simulink model "carsim_test2017"  (R2017b)
settings: Solver=FixedStepAuto  StartTime=0.0  StopTime=20  FixedStep=0.001  RelTol=1e-3
undefined symbols (not defined in the file or in its folder): ACC_MAP, ACC_MAP_ACCPEDL_BPY, ACC_MAP_REFSPD_BPX, BRK_MAP, BRK_MAP_BRKPEDL_BPX, ConvGear, CORNERING_STIFFNESS_APT, DIST_FR_AXLE_TO_CG_NVV, DIST_RE_AXLE_TO_CG_NVV, Fz, Fz_BPX, geartar, HYD_RATIO_APT, HYDRATIO_REFSPD_BPX, REFSPD_Q, REFSPD_R_LGT, REFSPD_R_WHL, STATIC_SPD, STATIC_TIME, VEHICLE_MASS_NVV, VEHICLE_YAW_INERTIA_NVV
libraries: simulink x22, simulink_extras x2, Solver_SF x1, SignalEditorBlockLib x1
(part 1 of 2)
settings Model: SimulationMode=accelerator  Creator=Ecoking  LastModifiedBy=Ecoking
settings DataIOCC: ReturnWorkspaceOutputs=on
settings DebuggingCC: UnconnectedInputMsg=none  UnconnectedOutputMsg=none  UnconnectedLineMsg=none
settings ModelReferenceCC: EnableRefExpFcnMdlSchedulingChecks=off
settings SFSimCC: SimUseLocalCustomCode=on
settings RTWCC: Description=Generic Real-Time Target  RTWUseLocalCustomCode=on

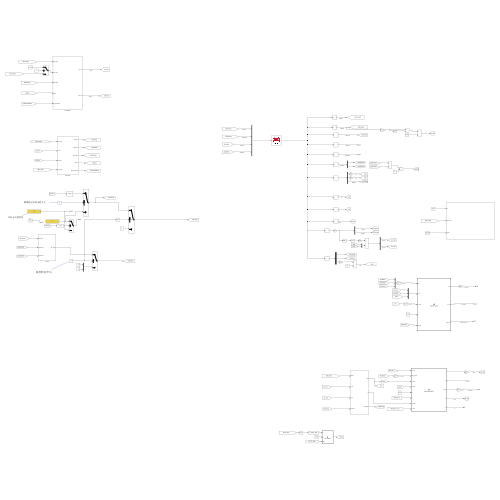
[thumbnail: Simulink's stored preview of the top-level diagram]
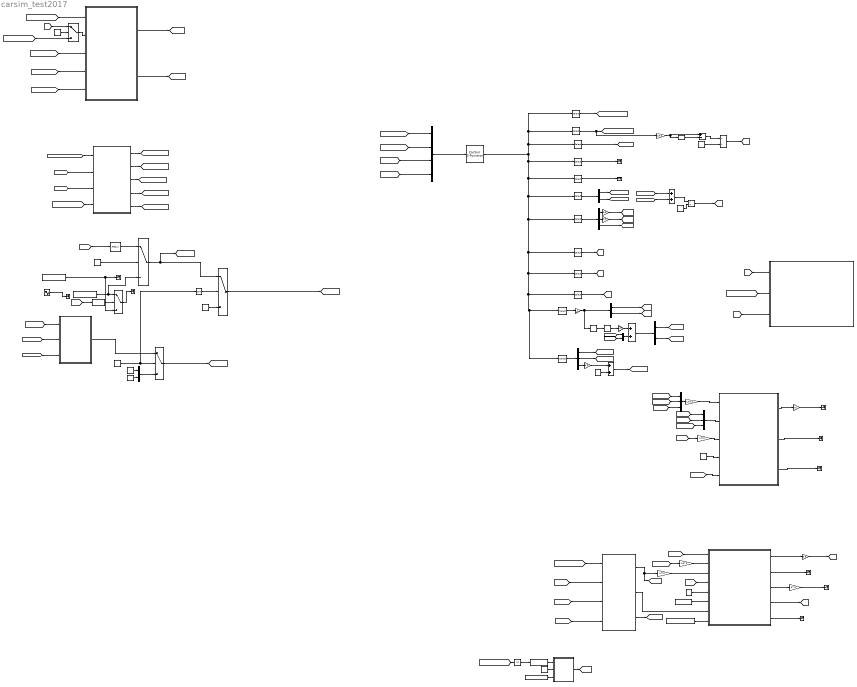
== system carsim_test2017 ==
  note: 线控转向开关
  note: 横摆稳定控制功能开关
  note: 目标方向盘转角
  Abs1 : Abs
  Add : Sum
  Add1 : Sum  Inputs=+-
  Add2 : Sum
  Add4 : Sum
  Asin : Trigonometry
  CarSim S-Function : Solver_SF/CarSim S-Function  Priority=1  SIMFILE=simfile.sim  Run_RTs=off  vs_state_ind=Run  StopMode_ind=Vehicle Model
  Compare To Constant2 : simulink/Logic and Bit Operations/Compare To Constant  relop=<=  const=STATIC_SPD  OutDataTypeStr=boolean
  Compare To Constant3 : simulink/Logic and Bit Operations/Compare To Constant  relop=<=  const=0.01  OutDataTypeStr=boolean
  Constant : Constant  Value=2
  Constant{1,11..14,25..26} (7 alike) : Constant  Value=0
  Constant{3,6..7,15} (4 alike) : Constant  Value=0.001
  Constant2 : Constant  Value=50
  Constant23 : Constant  Value=STATIC_TIME
  Constant24 : Constant  Value=REFSPD_R_LGT
  Constant4 : Constant  Value=REFSPD_Q
  Constant5 : Constant  Value=9.8
  Degrees to Radians : simulink_extras/Transformations/Degrees to Radians
  Delay : Delay  SampleTime=0.001
  Demux : Demux  Outputs=2
  Demux1 : Demux  Outputs=3
  Demux2 : Demux  Outputs=3
  Demux3 : Demux  Outputs=2
  Demux4 : Demux  Outputs=2
  Divide : Product  Inputs=*/
  Divide1 : Product  Inputs=*/
  Drv & Brk : Subsystem
  Gain{,1,6,9} (4 alike) : Gain  Gain=9.8
  Gain10 : Gain  Gain=1/3.6
  Gain11 : Gain  Gain=3.6
  Gain12 : Gain  Gain=1/57.3
  Gain2 : Gain  Gain=1/3.6
  Gain3 : Gain  Gain=3.6
  Gain4 : Gain  Gain=1/3.6
  Gain5 : Gain  Gain=-1
  Gain7 : Gain  Gain=57.3
  Gain8 : Gain  Gain=1/57.3
  Logical Operator : Logic  Operator=NOT  AllPortsSameDT=off  OutDataTypeStr=boolean
  MATLAB Function : MATLAB Function  TreatAsAtomicUnit=on
  MATLAB Function1 : MATLAB Function  TreatAsAtomicUnit=on
  MATLAB Function2 : MATLAB Function  TreatAsAtomicUnit=on
  Mux : Mux  Inputs=2
  Mux1 : Mux  Inputs=3
  Mux2 : Mux  Inputs=3
  Mux4 : Mux
  Mux9 : Mux  Inputs=2
  PID Controller1 : simulink/Continuous/PID Controller  Controller=PID  Form=Parallel  TimeDomain=Continuous-time  SampleTime=-1  IntegratorMethod=Forward Euler  ControllerParametersSource=internal  P=-10  I=-100  D=0  N=100  UseFilter=on  TunerSelectOption=Transfer Function Based (PID Tuner App)  InitialConditionSource=internal  InitialConditionForIntegrator=0  InitialConditionForFilter=0  DifferentiatorICPrevScaledInput=0  ExternalReset=none  TrackingMode=off  Kt=1  LimitOutput=off  UpperSaturationLimit=inf  LowerSaturationLimit=-inf  LinearizeAsGain=on  AntiWindupMode=none  Kb=1  POutMin=[]  POutMax=[]  IOutMin=[]  IOutMax=[]  DOutMin=[]  DOutMax=[]  NOutMin=[]  NOutMax=[]  SumOutMin=[]  SumOutMax=[]  SaturationOutMin=[]  SaturationOutMax=[]  PParamMin=[]  PParamMax=[]  IParamMin=[]  IParamMax=[]  DParamMin=[]  DParamMax=[]  NParamMin=[]  NParamMax=[]  KbParamMin=[]  KbParamMax=[]  KtParamMin=[]  KtParamMax=[]  KbOutMin=[]  KbOutMax=[]  KtOutMin=[]  KtOutMax=[]  IntegratorOutMin=[]  IntegratorOutMax=[]  FilterOutMin=[]  FilterOutMax=[]  SumI1OutMin=[]  SumI1OutMax=[]  SumI2OutMin=[]  SumI2OutMax=[]  SumI3OutMin=[]  SumI3OutMax=[]  SumDOutMin=[]  SumDOutMax=[]  DifferentiatorOutMin=[]  DifferentiatorOutMax=[]  FilterDiffOutCoefMin=[]  FilterDiffOutCoefMax=[]  ReciprocalOutMin=[]  ReciprocalOutMax=[]  SumDenOutMin=[]  SumDenOutMax=[]  SumNumOutMin=[]  SumNumOutMax=[]  DivideOutMin=[]  DivideOutMax=[]  IntegratorContinuousStateAttributes=''  IntegratorStateMustResolveToSignalObject=off  IntegratorRTWStateStorageClass=Auto  FilterContinuousStateAttributes=''  FilterStateMustResolveToSignalObject=off  FilterRTWStateStorageClass=Auto  InitialConditionSetting=State (most efficient)
  Selector : Selector  IndexOptions=Index vector (dialog)  Indices=1  OutputSizes=1
  Selector1 : Selector  IndexOptions=Index vector (dialog)  Indices=[2:5]  OutputSizes=1
  Selector12 : Selector  IndexOptions=Index vector (dialog)  Indices=[32 33]  OutputSizes=1
  Selector13 : Selector  IndexOptions=Index vector (dialog)  Indices=[34:36]  OutputSizes=1
  Selector2 : Selector  IndexOptions=Index vector (dialog)  Indices=[6:9]  OutputSizes=1
  Selector3 : Selector  IndexOptions=Index vector (dialog)  Indices=[10:13]  OutputSizes=1
  Selector4 : Selector  IndexOptions=Index vector (dialog)  Indices=[18:19]  OutputSizes=1
  Selector5 : Selector  IndexOptions=Index vector (dialog)  Indices=[20:22]  OutputSizes=1
  Selector6 : Selector  IndexOptions=Index vector (dialog)  Indices=[14:17]  OutputSizes=1
  Selector7 : Selector  IndexOptions=Index vector (dialog)  Indices=[23:26]  OutputSizes=1
  Selector8 : Selector  IndexOptions=Index vector (dialog)  Indices=[27:30]  OutputSizes=1
  Selector9 : Selector  IndexOptions=Index vector (dialog)  Indices=31  OutputSizes=1
  Sine Wave : Sin  Amplitude=50  SampleTime=0
  Subsystem : Subsystem
  Subsystem1 : Subsystem
  Switch{1..2,4..5,7} (5 alike) : Switch  Criteria=u2 > Threshold
  TCS & ABS : Subsystem
  Terminator{,1..9,11} (11 alike) : Terminator
  线控转向 : Subsystem
  wires:
  CarSim S-Function/1 -> Selector5/1, Selector8/1, Selector9/1, Selector13/1, Selector12/1, Selector7/1, Selector4/1, Selector6/1, Selector3/1, Selector2/1, Selector1/1, Selector/1
  Selector1/1 -> Gain4/1, [SPD_WHL]  "SpdWhl"
  Selector2/1 -> [MotTqAct]  "MotTqAct"
  Selector3/1 -> Terminator1/1  "HydTqAct"
  Mux4/1 -> CarSim S-Function/1
  [YawRate] -> PID Controller1/1
  PID Controller1/1 -> Switch1/1
  Constant11/1 -> Logical Operator/1, Switch4/2
  Constant12/1 -> Switch2/3
  Mux9/1 -> Switch4/3
  Switch4/1 -> [AgWhlTar]
  Constant13/1 -> Mux9/1
  Constant14/1 -> Mux9/2
  [SPD_WHL] -> TCS & ABS/1(SPD_WHL)
  [SPD_VEH] -> Switch5/3
  [MotTqDmd] -> TCS & ABS/3(MotTqDmd)
  Switch2/1 -> [SteerTar]
  Logical Operator/1 -> Switch2/2
  Switch1/1 -> [SteerDmd], Switch2/1
  Constant1/1 -> Switch1/2
  Constant2/1 -> Switch7/3, Terminator3/1
  [SteerDmd] -> 线控转向/1(SteerDmd)
  线控转向/1(pid_agwhl) -> Switch4/1
  [AgWhlActFl] -> 线控转向/2(AgWhlActFl)
  [AgWhlActFr] -> 线控转向/3(AgWhlActFr)
  Selector/1 -> [SPD_VEH]  "SpdVeh"
  Selector4/1 -> Demux/1  "AgWhlAct"
  Demux/1 -> [AgWhlActFl]
  Demux/2 -> [AgWhlActFr]
  [MotTqTar] -> Mux4/1  "MotTqTar"
  Selector6/1 -> Terminator2/1  "HydPbkAct"
  TCS & ABS/1(TcsLim) -> [TcsLim]  "TcsLim"
  [TcsLim] -> Drv & Brk/2(TcsLim)
  [SPD_VEH] -> Drv & Brk/1(SPD_VEH)
  [SPD_WHL] -> Drv & Brk/4(SPD_WHL)
  [AbsLim] -> Drv & Brk/3(MabsLim)
  Drv & Brk/1(MotTqTar) -> [MotTqTar]
  [HydPbkTar] -> Mux4/2  "HydPbkTar"
  [AgWhlTar] -> Mux4/4  "AgWhlTar"
  [SteerTar] -> Mux4/3  "SteerTar"
  Drv & Brk/2(HydPbkTar) -> [HydPbkTar]
  Drv & Brk/3(MotTqDmd) -> [MotTqDmd]
  Drv & Brk/4(Rgear) -> [Rgear]
  [Rgear] -> TCS & ABS/4(Rgear)
  Drv & Brk/5(BrkTqTotalDmd) -> [BrkTqTotalDmd]
  [BrkTqTotalDmd] -> TCS & ABS/5(BrkTqTotalDmd)
  TCS & ABS/2(AbsLim) -> [AbsLim]  "AbsLim"
  Selector5/1 -> Demux1/1
  Demux1/3 -> [YawRate]  "YawRate"
  Demux1/1 -> Gain/1
  Gain/1 -> [Lgt]  "Lgt"
  Demux1/2 -> Gain1/1
  Gain1/1 -> [Lat]  "Lat"
  Selector7/1 -> [Fz]  "Fz"
  Selector8/1 -> [Fy]  "Fy"
  Selector9/1 -> [Steer]  "Steer"
  [Fz] -> Subsystem/1(Fz)
  [SPD_VEH] -> Subsystem/2(SPD_VEH)
  [AgWhlActFl] -> Add/1
  [AgWhlActFr] -> Add/2
  Add/1 -> Divide/1
  Constant/1 -> Divide/2
  Divide/1 -> [whlag]
  [whlag] -> Subsystem/3(agwhl)
  Sine Wave/1 -> Terminator4/1
  [SPD_WHL] -> Subsystem1/1(Spdwhl)
  Subsystem1/1(Spd) -> [zv], Gain2/1  "zv"
  MATLAB Function/1(v) -> Gain3/1
  MATLAB Function/5(P) -> Terminator6/1  "P"
  MATLAB Function/3(theta) -> Gain7/1
  Gain3/1 -> [v_est]  "v_est"
  Delay/1 -> Add1/2
  Add1/1 -> Divide1/1
  Constant6/1 -> Divide1/2
  Divide1/1 -> [a_whl]
  Gain4/1 -> Delay/1, Add1/1
  Selector12/1 -> Gain5/1
  Gain5/1 -> Demux3/1, Degrees to Radians/1
  Degrees to Radians/1 -> Asin/1
  Asin/1 -> Gain6/1
  Gain6/1 -> Add4/1
  [Lgt] -> Mux/1
  Add4/1 -> Demux4/1
  Gain7/1 -> Terminator7/1  "theta_est"
  Selector13/1 -> Demux2/1
  Demux2/1 -> [PitchRate]
  Demux2/2 -> [RollRate]
  [PitchRate] -> Gain8/1
  [imu_lgt] -> MATLAB Function/1(a_meas)  "za"
  Gain8/1 -> MATLAB Function/2(omega_pitch)  "zp"
  Gain2/1 -> MATLAB Function/3(v_wheel)
  Constant3/1 -> MATLAB Function/5(dt)
  MATLAB Function/2(b) -> Terminator9/1  "b"
  Constant23/1 -> MATLAB Function1/3(delay)
  Constant15/1 -> MATLAB Function1/2(Ts)
  [SPD_VEH] -> Abs1/1
  Compare To Constant2/1 -> MATLAB Function1/1(u)
  Abs1/1 -> Compare To Constant2/1
  MATLAB Function1/1(y) -> [static]
  [static] -> MATLAB Function/4(is_static)
  Constant4/1 -> MATLAB Function/6(Q)
  Constant24/1 -> MATLAB Function/8(R_accel)
  MATLAB Function/4(a) -> [a_est]  "a_est"
  [v_est] -> Switch5/1
  Switch5/1 -> TCS & ABS/2(SPD_VEH)
  Constant25/1 -> Switch5/2
  [Agroad] -> Compare To Constant3/1
  Compare To Constant3/1 -> Switch7/2
  Constant26/1 -> Switch1/3, Switch7/1
  Switch7/1 -> Terminator11/1
  Subsystem1/2(R) -> MATLAB Function/7(R_wheel)
  [a_est] -> Subsystem1/3(a_est)
  [a_whl] -> Subsystem1/2(a_whl)
  [MotTqAct] -> Subsystem1/4(MotTqAct)
  Subsystem1/3(allSlipFlag) -> [allSlipFlag]
  Demux3/1 -> [Agroad]  "Agroad"
  Demux3/2 -> [RollSlop]  "RollSlop"
  [Lat] -> Mux/2
  Mux/1 -> Add4/2
  Demux4/1 -> [imu_lgt]  "imu_lgt"
  Demux4/2 -> [imu_lat]  "imu_lat"
  Demux2/3 -> Gain9/1
  Gain9/1 -> Add2/1
  Add2/1 -> [Vert]  "Vert"
  Constant5/1 -> Add2/2
  [RollRate] -> Mux1/1
  [YawRate] -> Mux1/3
  [PitchRate] -> Mux1/2
  Mux1/1 -> Gain12/1
  Mux2/1 -> MATLAB Function2/2(accel)
  [imu_lgt] -> Mux2/1
  [imu_lat] -> Mux2/2
  [Vert] -> Mux2/3
  [zv] -> Gain10/1
  Constant7/1 -> MATLAB Function2/4(dt)
  MATLAB Function2/1(v_car) -> Gain11/1
  [allSlipFlag] -> MATLAB Function2/5(slip_flag)
  Gain10/1 -> MATLAB Function2/3(v_wheel)
  Gain11/1 -> Terminator/1  "v_est_plus"
  Gain12/1 -> MATLAB Function2/1(gyro)
  MATLAB Function2/2(a_long) -> Terminator5/1  "a_est_plus"
  MATLAB Function2/3(pitch_deg) -> Terminator8/1  "theta_est_plus"

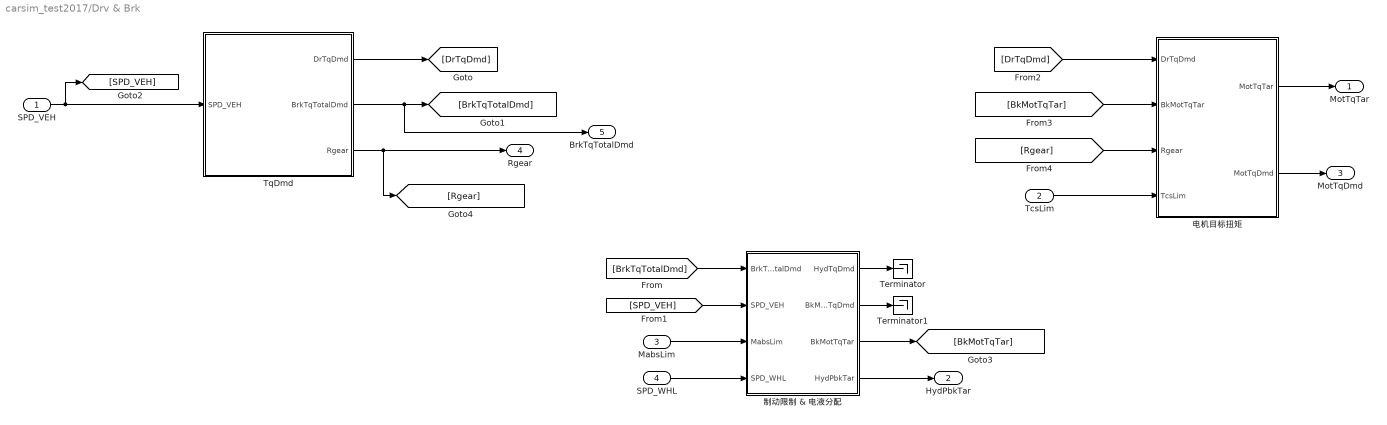
== system carsim_test2017/Drv & Brk ==
  SPD_VEH : Inport
  TcsLim : Inport  Port=2
  MabsLim : Inport  Port=3
  SPD_WHL : Inport  Port=4
  Terminator : Terminator
  Terminator1 : Terminator
  TqDmd : Subsystem
  制动限制 & 电液分配 : Subsystem
  电机目标扭矩 : Subsystem
  MotTqTar : Outport
  HydPbkTar : Outport  Port=2
  MotTqDmd : Outport  Port=3
  Rgear : Outport  Port=4
  BrkTqTotalDmd : Outport  Port=5
  wires:
  SPD_VEH/1 -> [SPD_VEH], TqDmd/1(SPD_VEH)
  TqDmd/3(Rgear) -> [Rgear], Rgear/1
  TqDmd/2(BrkTqTotalDmd) -> BrkTqTotalDmd/1, [BrkTqTotalDmd]
  TqDmd/1(DrTqDmd) -> [DrTqDmd]
  [BrkTqTotalDmd] -> 制动限制 & 电液分配/1(BrkTqTotalDmd)
  [SPD_VEH] -> 制动限制 & 电液分配/2(SPD_VEH)
  [DrTqDmd] -> 电机目标扭矩/1(DrTqDmd)
  [BkMotTqTar] -> 电机目标扭矩/2(BkMotTqTar)
  [Rgear] -> 电机目标扭矩/3(Rgear)
  TcsLim/1 -> 电机目标扭矩/4(TcsLim)
  MabsLim/1 -> 制动限制 & 电液分配/3(MabsLim)
  制动限制 & 电液分配/3(BkMotTqTar) -> [BkMotTqTar]
  SPD_WHL/1 -> 制动限制 & 电液分配/4(SPD_WHL)
  制动限制 & 电液分配/1(HydTqDmd) -> Terminator/1
  制动限制 & 电液分配/2(BkMotTqDmd) -> Terminator1/1
  制动限制 & 电液分配/4(HydPbkTar) -> HydPbkTar/1
  电机目标扭矩/1(MotTqTar) -> MotTqTar/1
  电机目标扭矩/2(MotTqDmd) -> MotTqDmd/1

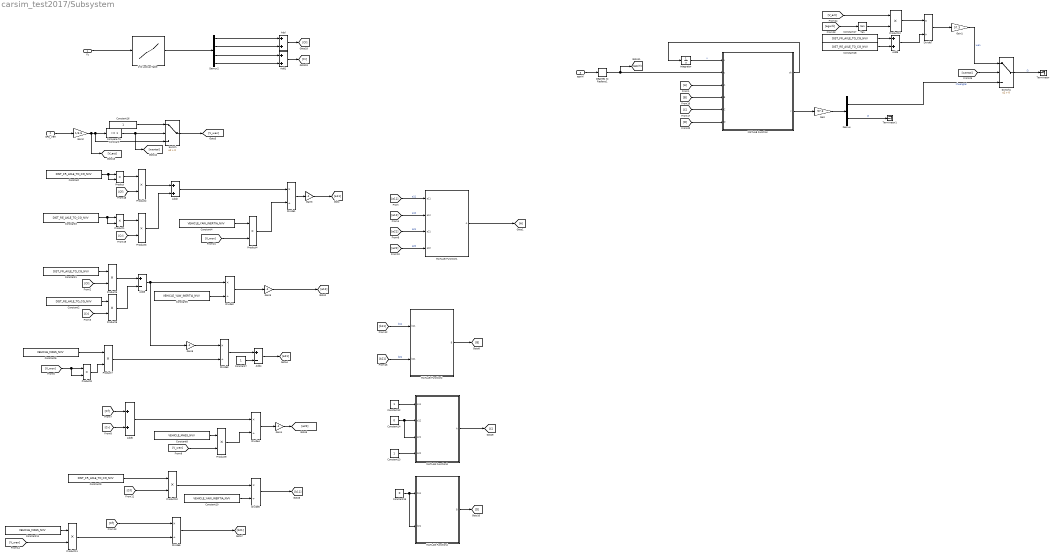
== system carsim_test2017/Subsystem ==
  Fz : Inport
  SPD_VEH : Inport  Port=2
  agwhl : Inport  Port=3
  2-D Lookup Table : Lookup_n-D  NumberOfTableDimensions=1  BreakpointsForDimension1=Fz_BPX  BreakpointsForDimension2=Fz  Table=CORNERING_STIFFNESS_APT  ExtrapMethod=Clip  UseLastTableValue=on  InternalRulePriority=Speed  RndMeth=Simplest  InputSameDT=on
  Add{,1..2,5..6} (5 alike) : Sum
  Add3 : Sum  Inputs=+-
  Add4 : Sum  Inputs=+-
  Compare To Constant : simulink/Logic and Bit Operations/Compare To Constant  relop=<=  const=1  OutDataTypeStr=boolean
  Constant{,1,9,17} (4 alike) : Constant  Value=DIST_FR_AXLE_TO_CG_NVV
  Constant10 : Constant  Value=VEHICLE_YAW_INERTIA_NVV
  Constant11 : Constant  Value=VEHICLE_MASS_NVV
  Constant{7,12..13,16} (4 alike) : Constant
  Constant14 : Constant  Value=0
  Constant15 : Constant  Value=0
  Constant18 : Constant  Value=DIST_RE_AXLE_TO_CG_NVV
  Constant2 : Constant  Value=DIST_RE_AXLE_TO_CG_NVV
  Constant3 : Constant  Value=DIST_RE_AXLE_TO_CG_NVV
  Constant4 : Constant  Value=VEHICLE_YAW_INERTIA_NVV
  Constant5 : Constant  Value=VEHICLE_YAW_INERTIA_NVV
  Constant6 : Constant  Value=VEHICLE_MASS_NVV
  Constant8 : Constant  Value=VEHICLE_MASS_NVV
  Degrees to Radians1 : simulink_extras/Transformations/Degrees to Radians
  Demux : Demux  Outputs=2
  Demux2 : Demux
  Divide{1..7} (7 alike) : Product  Inputs=*/
  Gain : Gain  Gain=57.3
  Gain1 : Gain  Gain=57.3
  Gain2 : Gain  Gain=1/3.6
  Gain{3..6} (4 alike) : Gain  Gain=-1
  Integrator : Integrator  InitialCondition=[0;0]
  MATLAB Function : MATLAB Function  TreatAsAtomicUnit=on
  MATLAB Function1 : MATLAB Function  TreatAsAtomicUnit=on
  MATLAB Function2 : MATLAB Function  TreatAsAtomicUnit=on
  MATLAB Function3 : MATLAB Function  TreatAsAtomicUnit=on
  MATLAB Function4 : MATLAB Function  TreatAsAtomicUnit=on
  Product{,1..12} (13 alike) : Product
  Switch : Switch  Criteria=u2 > Threshold
  Switch1 : Switch  Criteria=u2 > Threshold
  Tan : Trigonometry  Operator=tan
  Terminator : Terminator
  Terminator1 : Terminator
  wires:
  Constant4/1 -> Product4/1
  Constant/1 -> Product/2, Product/1
  Product2/1 -> Add2/1
  Product/1 -> Product2/1
  Add2/1 -> Divide1/1
  Constant3/1 -> Product1/2, Product1/1
  Degrees to Radians1/1 -> [agwhl], MATLAB Function/2(u)
  Product3/1 -> Add2/2
  Product1/1 -> Product3/1
  Divide1/1 -> Gain3/1
  Demux2/3 -> Add1/1
  SPD_VEH/1 -> Gain2/1
  [Cr] -> Product3/2
  Demux2/1 -> Add/1
  Demux2/4 -> Add1/2
  [Cf] -> Product2/2
  MATLAB Function1/1(A) -> [A]
  Fz/1 -> 2-D Lookup Table/1
  Demux2/2 -> Add/2
  agwhl/1 -> Degrees to Radians1/1
  [a11] -> MATLAB Function1/1(a11)  "a11"
  [A] -> MATLAB Function/3(A)
  Constant1/1 -> Product5/1
  [Cf] -> Product5/2
  Product5/1 -> Add3/1
  Constant2/1 -> Product6/1
  [Cr] -> Product6/2
  Product6/1 -> Add3/2
  Add3/1 -> Gain6/1, Divide2/1
  Constant5/1 -> Divide2/2
  Divide2/1 -> Gain5/1
  [a12] -> MATLAB Function1/2(a12)  "a12"
  Constant6/1 -> Product7/1
  [V_wen] -> Product8/2, Product8/1
  Product8/1 -> Product7/2
  Product7/1 -> Divide3/2
  Divide3/1 -> Add4/1
  Constant7/1 -> Add4/2
  Add4/1 -> [a21]
  [a21] -> MATLAB Function1/3(a21)  "a21"
  [Cf] -> Add5/1
  [Cr] -> Add5/2
  Add5/1 -> Divide4/1
  Constant8/1 -> Product9/1
  [V_wen] -> Product9/2
  Product9/1 -> Divide4/2
  Divide4/1 -> Gain4/1
  [a22] -> MATLAB Function1/4(a22)  "a22"
  [Cf] -> Product10/2
  Product10/1 -> Divide5/1
  Constant10/1 -> Divide5/2
  Divide5/1 -> [b11]
  [b11] -> MATLAB Function2/1(b11)  "b11"
  Constant9/1 -> Product10/1
  [Cf] -> Divide6/1
  [V_wen] -> Product11/2
  Constant11/1 -> Product11/1
  Product11/1 -> Divide6/2
  Divide6/1 -> [b21]
  [b21] -> MATLAB Function2/2(b21)  "b21"
  MATLAB Function2/1(B) -> [B]
  [B] -> MATLAB Function/4(B)
  Constant12/1 -> MATLAB Function3/1(a11)
  Constant13/1 -> MATLAB Function3/4(a22)
  Constant14/1 -> MATLAB Function3/3(a21), MATLAB Function3/2(a12)
  MATLAB Function3/1(A) -> [C]
  Constant15/1 -> MATLAB Function4/2(b21), MATLAB Function4/1(b11)
  MATLAB Function4/1(B) -> [D]
  [C] -> MATLAB Function/5(C)
  [D] -> MATLAB Function/6(D)
  MATLAB Function/2(y) -> Gain/1
  MATLAB Function/1(dx) -> Integrator/1
  Product4/1 -> Divide1/2
  Compare To Constant/1 -> Switch/2, [wentai]
  Gain2/1 -> [V_act], Switch/3, Compare To Constant/1
  Constant16/1 -> Switch/1
  Switch/1 -> [V_wen]
  [V_wen] -> Product4/2
  Integrator/1 -> MATLAB Function/1(x)  "x"
  Gain3/1 -> [a11]
  Gain4/1 -> [a22]
  Gain5/1 -> [a12]
  Gain6/1 -> Divide3/1
  Add/1 -> [Cf]
  Add1/1 -> [Cr]
  Gain/1 -> Demux/1
  2-D Lookup Table/1 -> Demux2/1
  Demux/1 -> Switch1/3  "zhuangtai"
  Demux/2 -> Terminator1/1  "β"
  [agwhl] -> Tan/1
  Tan/1 -> Product12/2
  [V_act] -> Product12/1
  Product12/1 -> Divide7/1
  Constant17/1 -> Add6/1
  Constant18/1 -> Add6/2
  Add6/1 -> Divide7/2
  Divide7/1 -> Gain1/1
  Gain1/1 -> Switch1/1  "wen"
  [wentai] -> Switch1/2
  Switch1/1 -> Terminator/1  "Ω"

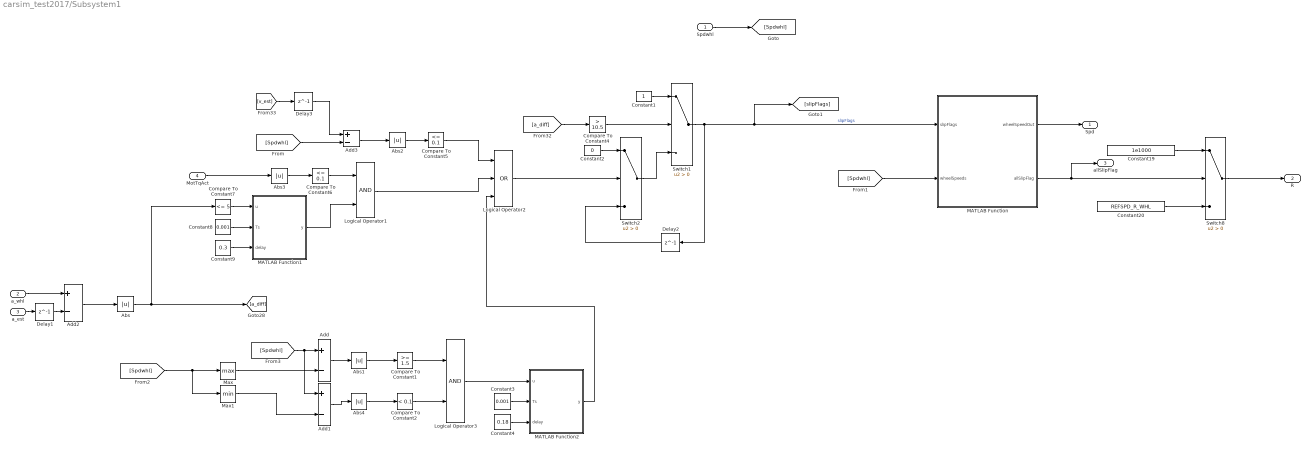
== system carsim_test2017/Subsystem1 ==
  Spdwhl : Inport
  a_whl : Inport  Port=2
  a_est : Inport  Port=3
  MotTqAct : Inport  Port=4
  Abs{,1..4} (5 alike) : Abs
  Add{,1..3} (4 alike) : Sum  Inputs=+-
  Compare To Constant1 : simulink/Logic and Bit Operations/Compare To Constant  relop=>=  const=1.5  OutDataTypeStr=boolean
  Compare To Constant2 : simulink/Logic and Bit Operations/Compare To Constant  relop=<  const=0.1  OutDataTypeStr=boolean
  Compare To Constant4 : simulink/Logic and Bit Operations/Compare To Constant  relop=>  const=10.5  OutDataTypeStr=boolean
  Compare To Constant5 : simulink/Logic and Bit Operations/Compare To Constant  relop=<=  const=0.1  OutDataTypeStr=boolean
  Compare To Constant6 : simulink/Logic and Bit Operations/Compare To Constant  relop=<=  const=0.1  OutDataTypeStr=boolean
  Compare To Constant7 : simulink/Logic and Bit Operations/Compare To Constant  relop=<=  const=5  OutDataTypeStr=boolean
  Constant1 : Constant
  Constant19 : Constant  Value=1e1000
  Constant2 : Constant  Value=0
  Constant20 : Constant  Value=REFSPD_R_WHL
  Constant3 : Constant  Value=0.001
  Constant4 : Constant  Value=0.18
  Constant8 : Constant  Value=0.001
  Constant9 : Constant  Value=0.3
  Delay1 : Delay  DelayLength=1
  Delay2 : Delay  DelayLength=1
  Delay3 : Delay  DelayLength=1
  Logical Operator1 : Logic  AllPortsSameDT=off  OutDataTypeStr=boolean
  Logical Operator2 : Logic  Operator=OR  Inputs=3  AllPortsSameDT=off  OutDataTypeStr=boolean
  Logical Operator3 : Logic  AllPortsSameDT=off  OutDataTypeStr=boolean
  MATLAB Function : MATLAB Function  TreatAsAtomicUnit=on
  MATLAB Function1 : MATLAB Function  TreatAsAtomicUnit=on
  MATLAB Function2 : MATLAB Function  TreatAsAtomicUnit=on
  Max : MinMax  Function=max
  Max1 : MinMax
  Switch1 : Switch  Criteria=u2 > Threshold
  Switch2 : Switch  Criteria=u2 > Threshold
  Switch8 : Switch  Criteria=u2 > Threshold
  Spd : Outport
  R : Outport  Port=2
  allSlipFlag : Outport  Port=3
  wires:
  Logical Operator1/1 -> Logical Operator2/2
  Abs3/1 -> Compare To Constant6/1
  Constant9/1 -> MATLAB Function1/3(delay)
  [v_est] -> Delay3/1
  a_whl/1 -> Add2/1
  Compare To Constant7/1 -> MATLAB Function1/1(u)
  Add3/1 -> Abs2/1
  Constant19/1 -> Switch8/1
  Compare To Constant6/1 -> Logical Operator1/1
  Abs2/1 -> Compare To Constant5/1
  a_est/1 -> Delay1/1
  MotTqAct/1 -> Abs3/1
  Constant8/1 -> MATLAB Function1/2(Ts)
  Add2/1 -> Abs/1
  Abs/1 -> Compare To Constant7/1, [a_diff]
  Logical Operator2/1 -> Switch2/2
  MATLAB Function1/1(y) -> Logical Operator1/2
  Delay3/1 -> Add3/1
  Compare To Constant5/1 -> Logical Operator2/1
  Spdwhl/1 -> [Spdwhl]
  [Spdwhl] -> Add3/2
  [Spdwhl] -> MATLAB Function/2(wheelSpeeds)
  [a_diff] -> Compare To Constant4/1
  Compare To Constant4/1 -> Switch1/2
  Switch2/1 -> Switch1/3
  Constant1/1 -> Switch1/1
  Switch1/1 -> [slipFlags], MATLAB Function/1(slipFlags), Delay2/1  "slipFlags"
  Delay2/1 -> Switch2/3
  Constant2/1 -> Switch2/1
  Switch8/1 -> R/1
  Constant20/1 -> Switch8/3
  MATLAB Function/1(wheelSpeedOut) -> Spd/1
  MATLAB Function/2(allSlipFlag) -> allSlipFlag/1, Switch8/2
  Delay1/1 -> Add2/2
  [Spdwhl] -> Max1/1, Max/1
  [Spdwhl] -> Add1/1, Add/1
  Max/1 -> Add/2
  Add/1 -> Abs1/1
  Abs1/1 -> Compare To Constant1/1
  Max1/1 -> Add1/2
  Add1/1 -> Abs4/1
  Abs4/1 -> Compare To Constant2/1
  Compare To Constant1/1 -> Logical Operator3/1
  Compare To Constant2/1 -> Logical Operator3/2
  Logical Operator3/1 -> MATLAB Function2/1(u)
  Constant3/1 -> MATLAB Function2/2(Ts)
  Constant4/1 -> MATLAB Function2/3(delay)
  MATLAB Function2/1(y) -> Logical Operator2/3

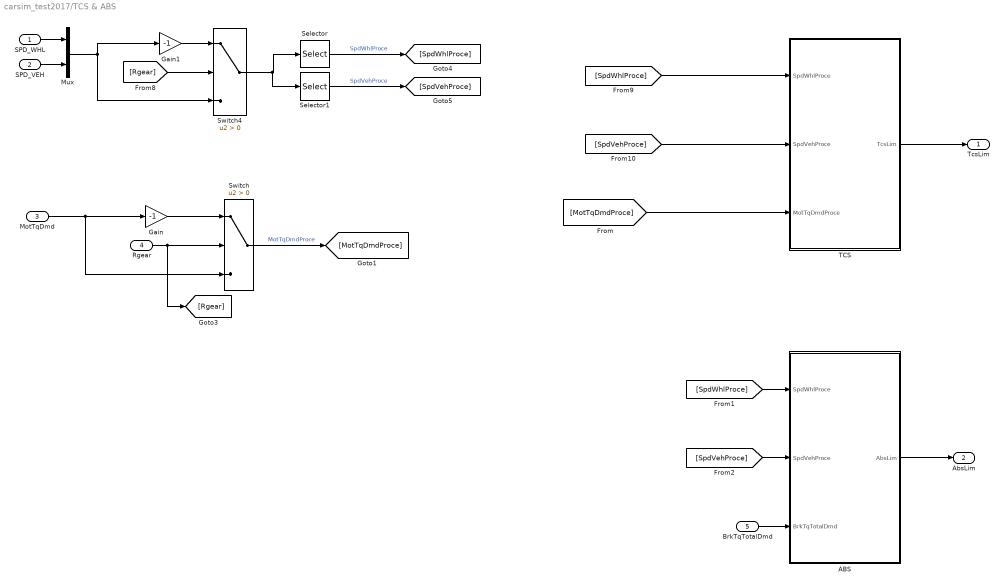
== system carsim_test2017/TCS & ABS ==
  SPD_WHL : Inport
  SPD_VEH : Inport  Port=2
  MotTqDmd : Inport  Port=3
  Rgear : Inport  Port=4
  BrkTqTotalDmd : Inport  Port=5
  ABS : Subsystem
  Gain : Gain  Gain=-1
  Gain1 : Gain  Gain=-1
  Mux : Mux  Inputs=2
  Selector : Selector  InputPortWidth=5  IndexOptions=Index vector (dialog)  Indices=[1:4]  OutputSizes=1
  Selector1 : Selector  InputPortWidth=5  IndexOptions=Index vector (dialog)  Indices=5  OutputSizes=1
  Switch : Switch  Criteria=u2 > Threshold
  Switch4 : Switch  Criteria=u2 > Threshold
  TCS : Subsystem
  TcsLim : Outport
  AbsLim : Outport  Port=2
  wires:
  MotTqDmd/1 -> Switch/3, Gain/1
  Rgear/1 -> [Rgear], Switch/2
  Gain/1 -> Switch/1
  Switch/1 -> [MotTqDmdProce]  "MotTqDmdProce"
  [Rgear] -> Switch4/2
  SPD_WHL/1 -> Mux/1
  SPD_VEH/1 -> Mux/2
  Mux/1 -> Switch4/3, Gain1/1
  Gain1/1 -> Switch4/1
  Switch4/1 -> Selector1/1, Selector/1
  Selector/1 -> [SpdWhlProce]  "SpdWhlProce"
  Selector1/1 -> [SpdVehProce]  "SpdVehProce"
  [SpdWhlProce] -> TCS/1(SpdWhlProce)
  [SpdVehProce] -> TCS/2(SpdVehProce)
  [MotTqDmdProce] -> TCS/3(MotTqDmdProce)
  TCS/1(TcsLim) -> TcsLim/1
  BrkTqTotalDmd/1 -> ABS/3(BrkTqTotalDmd)
  ABS/1(AbsLim) -> AbsLim/1
  [SpdWhlProce] -> ABS/1(SpdWhlProce)
  [SpdVehProce] -> ABS/2(SpdVehProce)

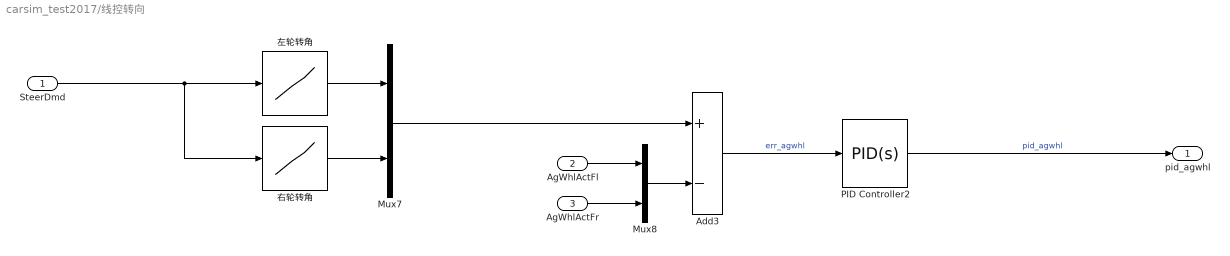
== system carsim_test2017/线控转向 ==
  SteerDmd : Inport
  AgWhlActFl : Inport  Port=2
  AgWhlActFr : Inport  Port=3
  Add3 : Sum  Inputs=+-
  Mux7 : Mux  Inputs=2
  Mux8 : Mux  Inputs=2
  PID Controller2 : simulink/Continuous/PID Controller  Controller=PID  Form=Parallel  TimeDomain=Continuous-time  SampleTime=-1  IntegratorMethod=Forward Euler  ControllerParametersSource=internal  P=0.3  I=10  D=0  N=100  UseFilter=on  TunerSelectOption=Transfer Function Based (PID Tuner App)  InitialConditionSource=internal  InitialConditionForIntegrator=0  InitialConditionForFilter=0  DifferentiatorICPrevScaledInput=0  ExternalReset=none  TrackingMode=off  Kt=1  LimitOutput=off  UpperSaturationLimit=inf  LowerSaturationLimit=-inf  LinearizeAsGain=on  AntiWindupMode=none  Kb=1  POutMin=[]  POutMax=[]  IOutMin=[]  IOutMax=[]  DOutMin=[]  DOutMax=[]  NOutMin=[]  NOutMax=[]  SumOutMin=[]  SumOutMax=[]  SaturationOutMin=[]  SaturationOutMax=[]  PParamMin=[]  PParamMax=[]  IParamMin=[]  IParamMax=[]  DParamMin=[]  DParamMax=[]  NParamMin=[]  NParamMax=[]  KbParamMin=[]  KbParamMax=[]  KtParamMin=[]  KtParamMax=[]  KbOutMin=[]  KbOutMax=[]  KtOutMin=[]  KtOutMax=[]  IntegratorOutMin=[]  IntegratorOutMax=[]  FilterOutMin=[]  FilterOutMax=[]  SumI1OutMin=[]  SumI1OutMax=[]  SumI2OutMin=[]  SumI2OutMax=[]  SumI3OutMin=[]  SumI3OutMax=[]  SumDOutMin=[]  SumDOutMax=[]  DifferentiatorOutMin=[]  DifferentiatorOutMax=[]  FilterDiffOutCoefMin=[]  FilterDiffOutCoefMax=[]  ReciprocalOutMin=[]  ReciprocalOutMax=[]  SumDenOutMin=[]  SumDenOutMax=[]  SumNumOutMin=[]  SumNumOutMax=[]  DivideOutMin=[]  DivideOutMax=[]  IntegratorContinuousStateAttributes=''  IntegratorStateMustResolveToSignalObject=off  IntegratorRTWStateStorageClass=Auto  FilterContinuousStateAttributes=''  FilterStateMustResolveToSignalObject=off  FilterRTWStateStorageClass=Auto  InitialConditionSetting=State (most efficient)
  右轮转角 : Lookup_n-D  NumberOfTableDimensions=1  BreakpointsForDimension1=|  BreakpointsForDimension2=[1:3]  Table=|  InternalRulePriority=Speed  RndMeth=Simplest  InputSameDT=on
      BreakpointsForDimension1=|
      | [-611.9673617
      | -605.8476881
      | -599.7280145
      | -593.6083409
      | -587.4886673
      | -581.3689937
      | -575.24932
      | -569.1296464
      | -563.0099728
      | -556.8902992
      | -550.7706256
      | -544.6509519
      | -538.5312783
      | -532.4116047
      | -526.2919311
      | -520.1722575
      | -514.0525839
      | -507.9329102
      | -501.8132366
      | -495.693563
      | -489.5738894
      | -483.4542158
      | -477.3345422
      | -471.2148685
      | -465.0951949
      | -458.9755213
      | -452.8558477
      | -446.7361741
      | -440.6165005
      | -434.4968268
      | -428.3771532
      | -422.2574796
      | -416.137806
      | -410.0181324
      | -403.8984587
      | -397.7787851
      | -391.6591115
      | -385.5394379
      | -379.4197643
      | -373.3000907
      | -367.180417
      | -361.0607434
      | -354.9410698
      | -348.8213962
      | -342.7017226
      | -336.582049
      | -330.4623753
      | -324.3427017
      | -318.2230281
      | -312.1033545
      | -305.9836809
      | -299.8640073
      | -293.7443336
      | -287.62466
      | -281.5049864
      | -275.3853128
      | -269.2656392
      | -263.1459655
      | -257.0262919
      | -250.9066183
      | -244.7869447
      | -238.6672711
      | -232.5475975
      | -226.4279238
      | -220.3082502
      | -214.1885766
      | -208.068903
      | -201.9492294
      | -195.8295558
      | -189.7098821
      | -183.5902085
      | -177.4705349
      | -171.3508613
      | -165.2311877
      | -159.1115141
      | -152.9918404
      | -146.8721668
      | -140.7524932
      | -134.6328196
      | -128.513146
      | -122.3934723
      | -116.2737987
      | -110.1541251
      | -104.0344515
      | -97.91477788
      | -91.79510426
      | -85.67543064
      | -79.55575703
      | -73.43608341
      | -67.31640979
      | -61.19673617
      | -55.07706256
      | -48.95738894
      | -42.83771532
      | -36.7180417
      | -30.59836809
      | -24.47869447
      | -18.35902085
      | -12.23934723
      | -6.119673617
      | 0
      | 6.119673617
      | 12.23934723
      | 18.35902085
      | 24.47869447
      | 30.59836809
      | 36.7180417
      | 42.83771532
      | 48.95738894
      | 55.07706256
      | 61.19673617
      | 67.31640979
      | 73.43608341
      | 79.55575703
      | 85.67543064
      | 91.79510426
      | 97.91477788
      | 104.0344515
      | 110.1541251
      | 116.2737987
      | 122.3934723
      | 128.513146
      | 134.6328196
      | 140.7524932
      | 146.8721668
      | 152.9918404
      | 159.1115141
      | 165.2311877
      | 171.3508613
      | 177.4705349
      | 183.5902085
      | 189.7098821
      | 195.8295558
      | 201.9492294
      | 208.068903
      | 214.1885766
      | 220.3082502
      | 226.4279238
      | 232.5475975
      | 238.6672711
      | 244.7869447
      | 250.9066183
      | 257.0262919
      | 263.1459655
      | 269.2656392
      | 275.3853128
      | 281.5049864
      | 287.62466
      | 293.7443336
      | 299.8640073
      | 305.9836809
      | 312.1033545
      | 318.2230281
      | 324.3427017
      | 330.4623753
      | 336.582049
      | 342.7017226
      | 348.8213962
      | 354.9410698
      | 361.0607434
      | 367.180417
      | 373.3000907
      | 379.4197643
      | 385.5394379
      | 391.6591115
      | 397.7787851
      | 403.8984587
      | 410.0181324
      | 416.137806
      | 422.2574796
      | 428.3771532
      | 434.4968268
      | 440.6165005
      | 446.7361741
      | 452.8558477
      | 458.9755213
      | 465.0951949
      | 471.2148685
      | 477.3345422
      | 483.4542158
      | 489.5738894
      | 495.693563
      | 501.8132366
      | 507.9329102
      | 514.0525839
      | 520.1722575
      | 526.2919311
      | 532.4116047
      | 538.5312783
      | 544.6509519
      | 550.7706256
      | 556.8902992
      | 563.0099728
      | 569.1296464
      | 575.24932
      | 581.3689937
      | 587.4886673
      | 593.6083409
      | 599.7280145
      | 605.8476881
      | 611.9673617]
      Table=|
      | [-41.64492301
      | -41.11007683
      | -40.57845207
      | -40.05001364
      | -39.52472734
      | -39.0025598
      | -38.48347842
      | -37.96745133
      | -37.45444735
      | -36.94443593
      | -36.43738715
      | -35.93327164
      | -35.43206057
      | -34.93372561
      | -34.43823892
      | -33.94557309
      | -33.45570115
      | -32.96859651
      | -32.48423297
      | -32.00258468
      | -31.52362614
      | -31.04733214
      | -30.57367781
      | -30.10263854
      | -29.63418999
      | -29.16830809
      | -28.70496902
      | -28.24414918
      | -27.7858252
      | -27.32997393
      | -26.87657239
      | -26.42559784
      | -25.9770277
      | -25.53083956
      | -25.0870112
      | -24.64552056
      | -24.20634573
      | -23.76946495
      | -23.33485663
      | -22.90249928
      | -22.47237158
      | -22.04445235
      | -21.6187205
      | -21.19515509
      | -20.77373531
      | -20.35444044
      | -19.9372499
      | -19.52214321
      | -19.1091
      | -18.69810001
      | -18.28912308
      | -17.88214916
      | -17.47715829
      | -17.07413062
      | -16.67304639
      | -16.27388593
      | -15.87662968
      | -15.48125814
      | -15.08775194
      | -14.69609177
      | -14.30625842
      | -13.91823277
      | -13.53199577
      | -13.14752847
      | -12.76481199
      | -12.38382755
      | -12.00455642
      | -11.62697999
      | -11.25107969
      | -10.87683706
      | -10.50423369
      | -10.13325127
      | -9.763871547
      | -9.396076346
      | -9.029847569
      | -8.665167187
      | -8.302017245
      | -7.940379853
      | -7.580237193
      | -7.221571516
      | -6.864365136
      | -6.508600436
      | -6.154259862
      | -5.801325924
      | -5.449781196
      | -5.09960831
      | -4.75078996
      | -4.4033089
      | -4.057147939
      | -3.712289945
      | -3.368717839
      | -3.026414596
      | -2.685363245
      | -2.345546864
      | -2.006948582
      | -1.669551575
      | -1.333339065
      | -0.998294321
      | -0.664400653
      | -0.331641416
      | 0
      | 0.330540162
      | 0.659995602
      | 0.988382819
      | 1.315718277
      | 1.642018409
      | 1.96729962
      | 2.291578288
      | 2.614870765
      | 2.937193383
      | 3.258562449
      | 3.578994256
      | 3.898505077
      | 4.217111173
      | 4.534828795
      | 4.851674183
      | 5.167663571
      | 5.48281319
      | 5.797139268
      | 6.110658037
      | 6.423385732
      | 6.735338595
      | 7.046532879
      | 7.356984849
      | 7.666710789
      | 7.975726998
      | 8.284049803
      | 8.591695552
      | 8.898680627
      | 9.205021441
      | 9.510734443
      | 9.815836124
      | 10.12034302
      | 10.42427171
      | 10.72763884
      | 11.03046109
      | 11.33275522
      | 11.63453805
      | 11.93582646
      | 12.23663743
      | 12.53698798
      | 12.83689526
      | 13.13637647
      | 13.43544893
      | 13.73413005
      | 14.03243734
      | 14.33038845
      | 14.62800111
      | 14.92529321
      | 15.22228273
      | 15.51898783
      | 15.81542679
      | 16.11161804
      | 16.40758017
      | 16.70333195
      | 16.99889232
      | 17.29428038
      | 17.58951545
      | 17.88461703
      | 18.17960484
      | 18.47449881
      | 18.7693191
      | 19.06408611
      | 19.35882048
      | 19.65354313
      | 19.94827523
      | 20.24303824
      | 20.53785392
      | 20.83274432
      | 21.12773184
      | 21.42283918
      | 21.71808943
      | 22.01350601
      | 22.30911274
      | 22.60493383
      | 22.9009939
      | 23.19731803
      | 23.49393171
      | 23.79086093
      | 24.08813216
      | 24.38577239
      | 24.68380915
      | 24.98227051
      | 25.28118515
      | 25.58058235
      | 25.88049202
      | 26.18094475
      | 26.48197182
      | 26.78360526
      | 27.08587784
      | 27.38882313
      | 27.69247556
      | 27.99687041
      | 28.3020439
      | 28.60803319
      | 28.91487647
      | 29.22261297
      | 29.53128304
      | 29.84092821
      | 30.15159121
      | 30.46331605]
  左轮转角 : Lookup_n-D  NumberOfTableDimensions=1  BreakpointsForDimension1=|  BreakpointsForDimension2=[1:3]  Table=|  InternalRulePriority=Speed  RndMeth=Simplest  InputSameDT=on
      BreakpointsForDimension1=|
      | [-611.9673617
      | -605.8476881
      | -599.7280145
      | -593.6083409
      | -587.4886673
      | -581.3689937
      | -575.24932
      | -569.1296464
      | -563.0099728
      | -556.8902992
      | -550.7706256
      | -544.6509519
      | -538.5312783
      | -532.4116047
      | -526.2919311
      | -520.1722575
      | -514.0525839
      | -507.9329102
      | -501.8132366
      | -495.693563
      | -489.5738894
      | -483.4542158
      | -477.3345422
      | -471.2148685
      | -465.0951949
      | -458.9755213
      | -452.8558477
      | -446.7361741
      | -440.6165005
      | -434.4968268
      | -428.3771532
      | -422.2574796
      | -416.137806
      | -410.0181324
      | -403.8984587
      | -397.7787851
      | -391.6591115
      | -385.5394379
      | -379.4197643
      | -373.3000907
      | -367.180417
      | -361.0607434
      | -354.9410698
      | -348.8213962
      | -342.7017226
      | -336.582049
      | -330.4623753
      | -324.3427017
      | -318.2230281
      | -312.1033545
      | -305.9836809
      | -299.8640073
      | -293.7443336
      | -287.62466
      | -281.5049864
      | -275.3853128
      | -269.2656392
      | -263.1459655
      | -257.0262919
      | -250.9066183
      | -244.7869447
      | -238.6672711
      | -232.5475975
      | -226.4279238
      | -220.3082502
      | -214.1885766
      | -208.068903
      | -201.9492294
      | -195.8295558
      | -189.7098821
      | -183.5902085
      | -177.4705349
      | -171.3508613
      | -165.2311877
      | -159.1115141
      | -152.9918404
      | -146.8721668
      | -140.7524932
      | -134.6328196
      | -128.513146
      | -122.3934723
      | -116.2737987
      | -110.1541251
      | -104.0344515
      | -97.91477788
      | -91.79510426
      | -85.67543064
      | -79.55575703
      | -73.43608341
      | -67.31640979
      | -61.19673617
      | -55.07706256
      | -48.95738894
      | -42.83771532
      | -36.7180417
      | -30.59836809
      | -24.47869447
      | -18.35902085
      | -12.23934723
      | -6.119673617
      | 0
      | 6.119673617
      | 12.23934723
      | 18.35902085
      | 24.47869447
      | 30.59836809
      | 36.7180417
      | 42.83771532
      | 48.95738894
      | 55.07706256
      | 61.19673617
      | 67.31640979
      | 73.43608341
      | 79.55575703
      | 85.67543064
      | 91.79510426
      | 97.91477788
      | 104.0344515
      | 110.1541251
      | 116.2737987
      | 122.3934723
      | 128.513146
      | 134.6328196
      | 140.7524932
      | 146.8721668
      | 152.9918404
      | 159.1115141
      | 165.2311877
      | 171.3508613
      | 177.4705349
      | 183.5902085
      | 189.7098821
      | 195.8295558
      | 201.9492294
      | 208.068903
      | 214.1885766
      | 220.3082502
      | 226.4279238
      | 232.5475975
      | 238.6672711
      | 244.7869447
      | 250.9066183
      | 257.0262919
      | 263.1459655
      | 269.2656392
      | 275.3853128
      | 281.5049864
      | 287.62466
      | 293.7443336
      | 299.8640073
      | 305.9836809
      | 312.1033545
      | 318.2230281
      | 324.3427017
      | 330.4623753
      | 336.582049
      | 342.7017226
      | 348.8213962
      | 354.9410698
      | 361.0607434
      | 367.180417
      | 373.3000907
      | 379.4197643
      | 385.5394379
      | 391.6591115
      | 397.7787851
      | 403.8984587
      | 410.0181324
      | 416.137806
      | 422.2574796
      | 428.3771532
      | 434.4968268
      | 440.6165005
      | 446.7361741
      | 452.8558477
      | 458.9755213
      | 465.0951949
      | 471.2148685
      | 477.3345422
      | 483.4542158
      | 489.5738894
      | 495.693563
      | 501.8132366
      | 507.9329102
      | 514.0525839
      | 520.1722575
      | 526.2919311
      | 532.4116047
      | 538.5312783
      | 544.6509519
      | 550.7706256
      | 556.8902992
      | 563.0099728
      | 569.1296464
      | 575.24932
      | 581.3689937
      | 587.4886673
      | 593.6083409
      | 599.7280145
      | 605.8476881
      | 611.9673617]
      Table=|
      | [-30.46331605
      | -30.15159121
      | -29.84092821
      | -29.53128304
      | -29.22261297
      | -28.91487647
      | -28.60803319
      | -28.3020439
      | -27.99687041
      | -27.69247556
      | -27.38882313
      | -27.08587784
      | -26.78360526
      | -26.48197182
      | -26.18094475
      | -25.88049202
      | -25.58058235
      | -25.28118515
      | -24.98227051
      | -24.68380915
      | -24.38577239
      | -24.08813216
      | -23.79086093
      | -23.49393171
      | -23.19731803
      | -22.9009939
      | -22.60493383
      | -22.30911274
      | -22.01350601
      | -21.71808943
      | -21.42283918
      | -21.12773184
      | -20.83274432
      | -20.53785392
      | -20.24303824
      | -19.94827523
      | -19.65354313
      | -19.35882048
      | -19.06408611
      | -18.7693191
      | -18.47449881
      | -18.17960484
      | -17.88461703
      | -17.58951545
      | -17.29428038
      | -16.99889232
      | -16.70333195
      | -16.40758017
      | -16.11161804
      | -15.81542679
      | -15.51898783
      | -15.22228273
      | -14.92529321
      | -14.62800111
      | -14.33038845
      | -14.03243734
      | -13.73413005
      | -13.43544893
      | -13.13637647
      | -12.83689526
      | -12.53698798
      | -12.23663743
      | -11.93582646
      | -11.63453805
      | -11.33275522
      | -11.03046109
      | -10.72763884
      | -10.42427171
      | -10.12034302
      | -9.815836124
      | -9.510734443
      | -9.205021441
      | -8.898680627
      | -8.591695552
      | -8.284049803
      | -7.975726998
      | -7.666710789
      | -7.356984849
      | -7.046532879
      | -6.735338595
      | -6.423385732
      | -6.110658037
      | -5.797139268
      | -5.48281319
      | -5.167663571
      | -4.851674183
      | -4.534828795
      | -4.217111173
      | -3.898505077
      | -3.578994256
      | -3.258562449
      | -2.937193383
      | -2.614870765
      | -2.291578288
      | -1.96729962
      | -1.642018409
      | -1.315718277
      | -0.988382819
      | -0.659995602
      | -0.330540162
      | 0
      | 0.331641416
      | 0.664400653
      | 0.998294321
      | 1.333339065
      | 1.669551575
      | 2.006948582
      | 2.345546864
      | 2.685363245
      | 3.026414596
      | 3.368717839
      | 3.712289945
      | 4.057147939
      | 4.4033089
      | 4.75078996
      | 5.09960831
      | 5.449781196
      | 5.801325924
      | 6.154259862
      | 6.508600436
      | 6.864365136
      | 7.221571516
      | 7.580237193
      | 7.940379853
      | 8.302017245
      | 8.665167187
      | 9.029847569
      | 9.396076346
      | 9.763871547
      | 10.13325127
      | 10.50423369
      | 10.87683706
      | 11.25107969
      | 11.62697999
      | 12.00455642
      | 12.38382755
      | 12.76481199
      | 13.14752847
      | 13.53199577
      | 13.91823277
      | 14.30625842
      | 14.69609177
      | 15.08775194
      | 15.48125814
      | 15.87662968
      | 16.27388593
      | 16.67304639
      | 17.07413062
      | 17.47715829
      | 17.88214916
      | 18.28912308
      | 18.69810001
      | 19.1091
      | 19.52214321
      | 19.9372499
      | 20.35444044
      | 20.77373531
      | 21.19515509
      | 21.6187205
      | 22.04445235
      | 22.47237158
      | 22.90249928
      | 23.33485663
      | 23.76946495
      | 24.20634573
      | 24.64552056
      | 25.0870112
      | 25.53083956
      | 25.9770277
      | 26.42559784
      | 26.87657239
      | 27.32997393
      | 27.7858252
      | 28.24414918
      | 28.70496902
      | 29.16830809
      | 29.63418999
      | 30.10263854
      | 30.57367781
      | 31.04733214
      | 31.52362614
      | 32.00258468
      | 32.48423297
      | 32.96859651
      | 33.45570115
      | 33.94557309
      | 34.43823892
      | 34.93372561
      | 35.43206057
      | 35.93327164
      | 36.43738715
      | 36.94443593
      | 37.45444735
      | 37.96745133
      | 38.48347842
      | 39.0025598
      | 39.52472734
      | 40.05001364
      | 40.57845207
      | 41.11007683
      | 41.64492301]
  pid_agwhl : Outport
  wires:
  左轮转角/1 -> Mux7/1
  Mux7/1 -> Add3/1
  右轮转角/1 -> Mux7/2
  Add3/1 -> PID Controller2/1  "err_agwhl"
  AgWhlActFl/1 -> Mux8/1
  Mux8/1 -> Add3/2
  SteerDmd/1 -> 右轮转角/1, 左轮转角/1
  AgWhlActFr/1 -> Mux8/2
  PID Controller2/1 -> pid_agwhl/1  "pid_agwhl"

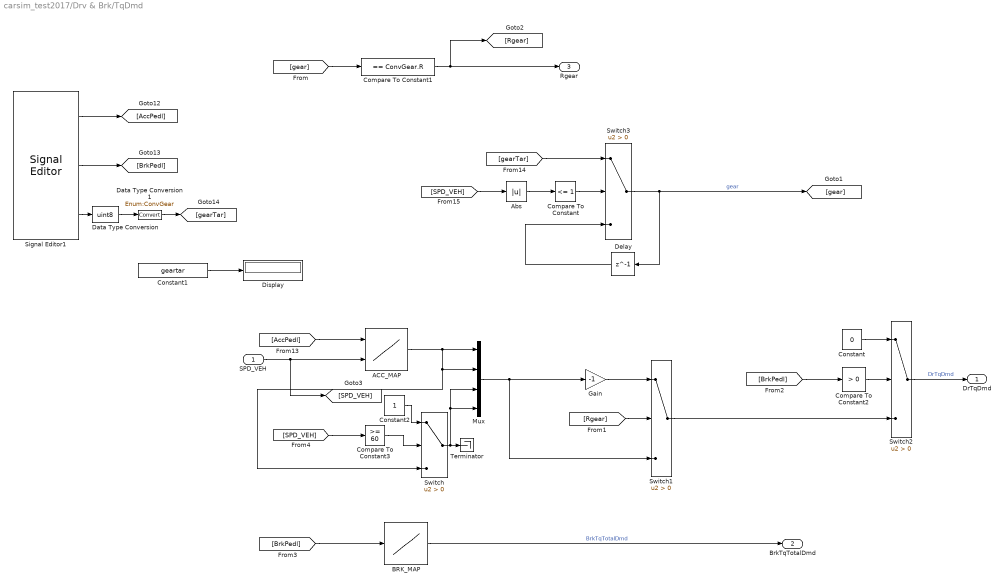
== system carsim_test2017/Drv & Brk/TqDmd ==
  SPD_VEH : Inport
  ACC_MAP : Lookup_n-D  BreakpointsForDimension1=ACC_MAP_ACCPEDL_BPY  BreakpointsForDimension2=ACC_MAP_REFSPD_BPX  Table=ACC_MAP  ExtrapMethod=Clip  UseLastTableValue=on  InternalRulePriority=Speed  RndMeth=Simplest  InputSameDT=on
  Abs : Abs
  BRK_MAP : Lookup_n-D  NumberOfTableDimensions=1  BreakpointsForDimension1=BRK_MAP_BRKPEDL_BPX  BreakpointsForDimension2=ACC_MAP_REFSPD_BPX  Table=BRK_MAP  ExtrapMethod=Clip  UseLastTableValue=on  InternalRulePriority=Speed  RndMeth=Simplest  InputSameDT=on
  Compare To Constant : simulink/Logic and Bit Operations/Compare To Constant  relop=<=  const=1  OutDataTypeStr=boolean
  Compare To Constant1 : simulink/Logic and Bit Operations/Compare To Constant  relop===  const=ConvGear.R  OutDataTypeStr=boolean
  Compare To Constant2 : simulink/Logic and Bit Operations/Compare To Constant  relop=>  const=0  OutDataTypeStr=boolean
  Compare To Constant3 : simulink/Logic and Bit Operations/Compare To Constant  relop=>=  const=60  OutDataTypeStr=boolean
  Constant : Constant  Value=0
  Constant1 : Constant  Value=geartar
  Constant2 : Constant
  Data Type Conversion : DataTypeConversion  OutDataTypeStr=uint8
  Data Type Conversion1 : DataTypeConversion  OutDataTypeStr=Enum:ConvGear
  Delay : Delay  DelayLength=1  InitialCondition=ConvGear.D
  Display : Display
  Gain : Gain  Gain=-1
  Mux : Mux
  Signal Editor1 : SignalEditorBlockLib/Signal Editor  FileName=D:\CarsimWorkspace\mdl\signaledit.mat  ActiveScenario=Scenario  ActiveSignal=AccPedl  IsBus=off  OutputBusObjectStr=Bus: BusObject  SampleTime=0  Interpolate=off  ZeroCross=off  OutputAfterFinalValue=Setting to zero  Unit=inherit
  Switch{,1..3} (4 alike) : Switch  Criteria=u2 > Threshold
  Terminator : Terminator
  DrTqDmd : Outport
  BrkTqTotalDmd : Outport  Port=2
  Rgear : Outport  Port=3
  wires:
  Data Type Conversion1/1 -> [gearTar]
  Data Type Conversion/1 -> Data Type Conversion1/1
  Signal Editor1/1 -> [AccPedl]
  Switch3/1 -> [gear], Delay/1  "gear"
  Signal Editor1/2 -> [BrkPedl]
  ACC_MAP/1 -> Switch/3, Mux/2, Mux/1
  Mux/1 -> Switch1/3, Gain/1
  [gearTar] -> Switch3/1
  Signal Editor1/3 -> Data Type Conversion/1
  Compare To Constant1/1 -> Rgear/1, [Rgear]
  [gear] -> Compare To Constant1/1
  [AccPedl] -> ACC_MAP/1
  [SPD_VEH] -> Abs/1
  [Rgear] -> Switch1/2
  Delay/1 -> Switch3/3
  Compare To Constant/1 -> Switch3/2
  SPD_VEH/1 -> [SPD_VEH], ACC_MAP/2
  Abs/1 -> Compare To Constant/1
  Gain/1 -> Switch1/1
  Switch1/1 -> Switch2/3
  Compare To Constant2/1 -> Switch2/2
  [BrkPedl] -> Compare To Constant2/1
  Switch2/1 -> DrTqDmd/1  "DrTqDmd"
  Constant/1 -> Switch2/1
  [BrkPedl] -> BRK_MAP/1
  BRK_MAP/1 -> BrkTqTotalDmd/1  "BrkTqTotalDmd"
  Constant1/1 -> Display/1
  [SPD_VEH] -> Compare To Constant3/1
  Compare To Constant3/1 -> Switch/2
  Constant2/1 -> Switch/1
  Switch/1 -> Mux/4, Mux/3, Terminator/1

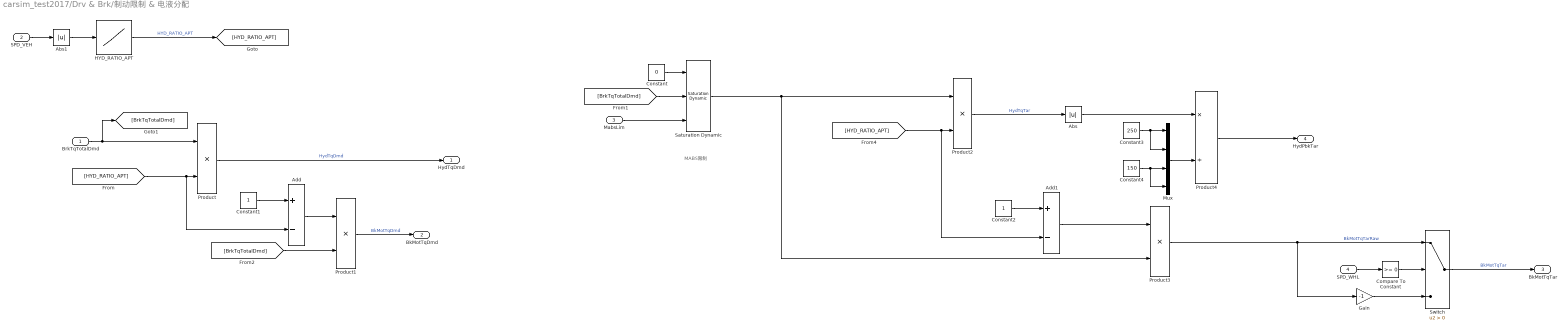
== system carsim_test2017/Drv & Brk/制动限制 & 电液分配 ==
  note: MABS限制
  BrkTqTotalDmd : Inport
  SPD_VEH : Inport  Port=2
  MabsLim : Inport  Port=3
  SPD_WHL : Inport  Port=4
  Abs : Abs
  Abs1 : Abs
  Add : Sum  Inputs=+-
  Add1 : Sum  Inputs=+-
  Compare To Constant : simulink/Logic and Bit Operations/Compare To Constant  relop=>=  const=0  OutDataTypeStr=boolean
  Constant : Constant  Value=0
  Constant1 : Constant
  Constant2 : Constant
  Constant3 : Constant  Value=250
  Constant4 : Constant  Value=150
  Gain : Gain  Gain=-1
  HYD_RATIO_APT : Lookup_n-D  NumberOfTableDimensions=1  BreakpointsForDimension1=HYDRATIO_REFSPD_BPX  BreakpointsForDimension2=[1:3]  Table=HYD_RATIO_APT  ExtrapMethod=Clip  UseLastTableValue=on  InternalRulePriority=Speed  RndMeth=Simplest  InputSameDT=on
  Mux : Mux
  Product{,1..3} (4 alike) : Product
  Product4 : Product  Inputs=*/
  Saturation Dynamic : simulink/Discontinuities/Saturation Dynamic  OutMin=[]  OutMax=[]  OutDataTypeStr=Inherit: Same as second input  OutDataType=fixdt(1, 16)  OutScaling=2^-10  DoSatur=off
  Switch : Switch  Criteria=u2 > Threshold
  HydTqDmd : Outport
  BkMotTqDmd : Outport  Port=2
  BkMotTqTar : Outport  Port=3
  HydPbkTar : Outport  Port=4
  wires:
  SPD_VEH/1 -> Abs1/1
  HYD_RATIO_APT/1 -> [HYD_RATIO_APT]  "HYD_RATIO_APT"
  [HYD_RATIO_APT] -> Add/2, Product/2
  BrkTqTotalDmd/1 -> Product/1, [BrkTqTotalDmd]
  MabsLim/1 -> Saturation Dynamic/3
  Constant/1 -> Saturation Dynamic/1
  [BrkTqTotalDmd] -> Saturation Dynamic/2
  Product/1 -> HydTqDmd/1  "HydTqDmd"
  Product1/1 -> BkMotTqDmd/1  "BkMotTqDmd"
  Constant1/1 -> Add/1
  [BrkTqTotalDmd] -> Product1/2
  Add/1 -> Product1/1
  Saturation Dynamic/1 -> Product3/2, Product2/1
  Add1/1 -> Product3/1
  Product2/1 -> Abs/1  "HydTqTar"
  Constant2/1 -> Add1/1
  [HYD_RATIO_APT] -> Add1/2, Product2/2
  Product3/1 -> Gain/1, Switch/1  "BkMotTqTarRaw"
  Compare To Constant/1 -> Switch/2
  SPD_WHL/1 -> Compare To Constant/1
  Switch/1 -> BkMotTqTar/1  "BkMotTqTar"
  Gain/1 -> Switch/3
  Constant3/1 -> Mux/2, Mux/1
  Constant4/1 -> Mux/3, Mux/4
  Product4/1 -> HydPbkTar/1
  Mux/1 -> Product4/2
  Abs/1 -> Product4/1
  Abs1/1 -> HYD_RATIO_APT/1

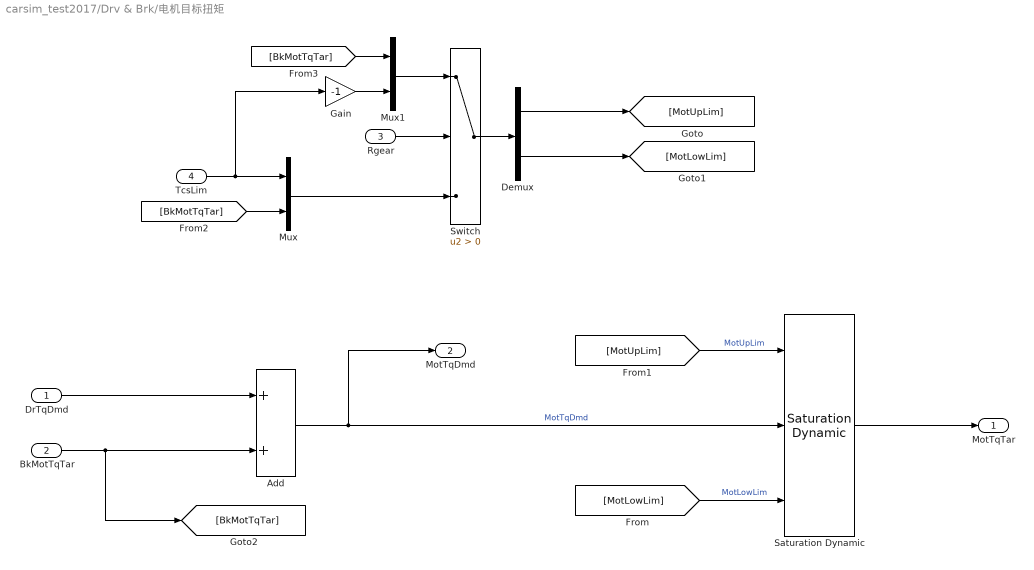
== system carsim_test2017/Drv & Brk/电机目标扭矩 ==
  DrTqDmd : Inport
  BkMotTqTar : Inport  Port=2
  Rgear : Inport  Port=3
  TcsLim : Inport  Port=4
  Add : Sum
  Demux : Demux  Outputs=2
  Gain : Gain  Gain=-1
  Mux : Mux  Inputs=2
  Mux1 : Mux  Inputs=2
  Saturation Dynamic : simulink/Discontinuities/Saturation Dynamic  OutMin=[]  OutMax=[]  OutDataTypeStr=Inherit: Same as second input  OutDataType=fixdt(1, 16)  OutScaling=2^-10  DoSatur=off
  Switch : Switch  Criteria=u2 > Threshold
  MotTqTar : Outport
  MotTqDmd : Outport  Port=2
  wires:
  DrTqDmd/1 -> Add/1
  BkMotTqTar/1 -> [BkMotTqTar], Add/2
  Add/1 -> Saturation Dynamic/2, MotTqDmd/1  "MotTqDmd"
  Rgear/1 -> Switch/2
  Mux/1 -> Switch/3
  TcsLim/1 -> Mux/1, Gain/1
  Switch/1 -> Demux/1
  Demux/1 -> [MotUpLim]
  Demux/2 -> [MotLowLim]
  [MotLowLim] -> Saturation Dynamic/3  "MotLowLim"
  [MotUpLim] -> Saturation Dynamic/1  "MotUpLim"
  Mux1/1 -> Switch/1
  [BkMotTqTar] -> Mux/2
  [BkMotTqTar] -> Mux1/1
  Saturation Dynamic/1 -> MotTqTar/1
  Gain/1 -> Mux1/2

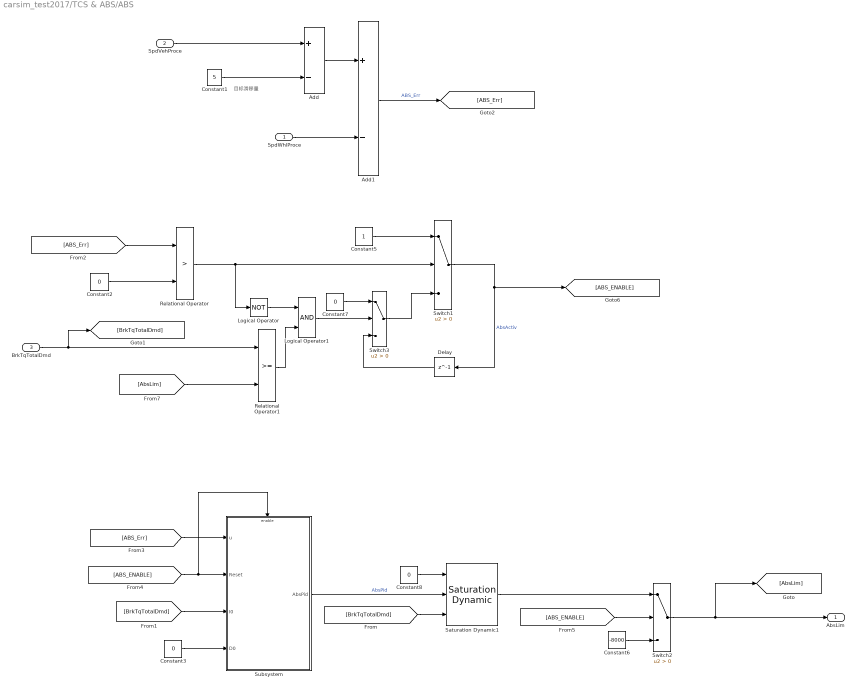
== system carsim_test2017/TCS & ABS/ABS ==
  note: 目标滑移量
  SpdWhlProce : Inport
  SpdVehProce : Inport  Port=2
  BrkTqTotalDmd : Inport  Port=3
  Add : Sum  Inputs=+-
  Add1 : Sum  Inputs=+-
  Constant1 : Constant  Value=5
  Constant{2..3,7..8} (4 alike) : Constant  Value=0
  Constant5 : Constant
  Constant6 : Constant  Value=-8000
  Delay : Delay  DelayLength=1
  Logical Operator : Logic  Operator=NOT  AllPortsSameDT=off  OutDataTypeStr=boolean
  Logical Operator1 : Logic  AllPortsSameDT=off  OutDataTypeStr=boolean
  Relational Operator : RelationalOperator  Operator=>  OutDataTypeStr=boolean  RndMeth=Simplest
  Relational Operator1 : RelationalOperator  OutDataTypeStr=boolean  RndMeth=Simplest
  Saturation Dynamic1 : simulink/Discontinuities/Saturation Dynamic  OutMin=[]  OutMax=[]  OutDataTypeStr=Inherit: Same as second input  OutDataType=fixdt(1, 16)  OutScaling=2^-10  DoSatur=off
  Subsystem : Subsystem
  Switch1 : Switch  Criteria=u2 > Threshold
  Switch2 : Switch  Criteria=u2 > Threshold
  Switch3 : Switch  Criteria=u2 > Threshold
  AbsLim : Outport
  wires:
  SpdVehProce/1 -> Add/1
  Constant3/1 -> Subsystem/4(D0)
  [BrkTqTotalDmd] -> Subsystem/3(I0)
  Saturation Dynamic1/1 -> Switch2/1
  Constant6/1 -> Switch2/3
  [ABS_Err] -> Relational Operator/1
  Constant7/1 -> Switch3/1
  [ABS_ENABLE] -> Switch2/2
  Relational Operator/1 -> Switch1/2, Logical Operator/1
  Subsystem/1(AbsPid) -> Saturation Dynamic1/2  "AbsPid"
  Relational Operator1/1 -> Logical Operator1/2
  BrkTqTotalDmd/1 -> Relational Operator1/1, [BrkTqTotalDmd]
  Delay/1 -> Switch3/3
  Constant1/1 -> Add/2
  Add1/1 -> [ABS_Err]  "ABS_Err"
  Logical Operator1/1 -> Switch3/2
  Switch3/1 -> Switch1/3
  Constant2/1 -> Relational Operator/2
  [AbsLim] -> Relational Operator1/2
  Add/1 -> Add1/1
  Logical Operator/1 -> Logical Operator1/1
  Switch2/1 -> [AbsLim], AbsLim/1
  [ABS_ENABLE] -> Subsystem/2(Reset), Subsystem/Enable
  Switch1/1 -> Delay/1, [ABS_ENABLE]  "AbsActiv"
  Constant5/1 -> Switch1/1
  [ABS_Err] -> Subsystem/1(u)
  SpdWhlProce/1 -> Add1/2
  Constant8/1 -> Saturation Dynamic1/1
  [BrkTqTotalDmd] -> Saturation Dynamic1/3
